simulink model "PURE_PURSUIT"  (R2022b)
settings: Solver=FixedStepAuto  StartTime=0.0  StopTime=400  FixedStep=0.1  RelTol=1e-3
InitFcn:
  | load('pure_pursuit_trajectory.mat');
values from neighbouring files (symbols this model uses):
  trajectory_matrix = trajectory_points    [MAIN_PURE_PURSUIT.m]
undefined symbols (not defined in the file or in its folder): debug_enabled
libraries: robotmobilelib x1
settings Model: Creator=emanuela  LastModifiedBy=emanuela
settings DataIOCC: ReturnWorkspaceOutputs=off

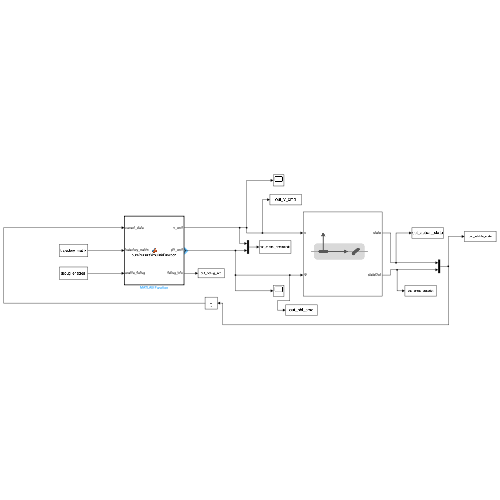
[thumbnail: Simulink's stored preview of the top-level diagram]
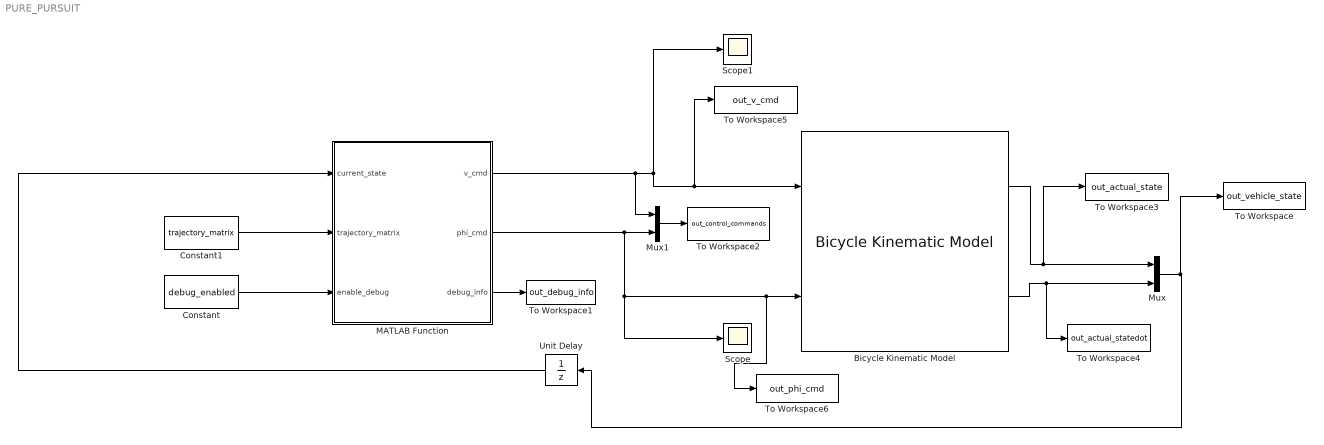
== system PURE_PURSUIT ==
  Bicycle Kinematic Model : robotmobilelib/Bicycle Kinematic Model  VehicleInputs=Vehicle Speed & Steering Angle  WheelBase=2.8  VehicleSpeedRange=[0 3]  MaxSteeringAngle=pi/4  InitialState=initialPose  SimulateUsing=Interpreted execution
  Constant : Constant  Value=debug_enabled
  Constant1 : Constant  Value=trajectory_matrix
  MATLAB Function : MATLAB Function  TreatAsAtomicUnit=on
  Mux : Mux  Inputs=2
  Mux1 : Mux  Inputs=2
  Scope : Scope
  Scope1 : Scope
  To Workspace : ToWorkspace  VariableName=out_vehicle_state  SaveFormat=Timeseries  SampleTime=-1
  To Workspace1 : ToWorkspace  VariableName=out_debug_info  SaveFormat=Timeseries  SampleTime=-1
  To Workspace2 : ToWorkspace  VariableName=out_control_commands  SaveFormat=Timeseries  SampleTime=-1
  To Workspace3 : ToWorkspace  VariableName=out_actual_state  SaveFormat=Timeseries  SampleTime=-1
  To Workspace4 : ToWorkspace  VariableName=out_actual_statedot  SaveFormat=Timeseries  SampleTime=-1
  To Workspace5 : ToWorkspace  VariableName=out_v_cmd  SaveFormat=Timeseries  SampleTime=-1
  To Workspace6 : ToWorkspace  VariableName=out_phi_cmd  SaveFormat=Timeseries  SampleTime=-1
  Unit Delay : UnitDelay  InitialCondition=[36.35,44.05,0,0,0,0]  SampleTime=0.1  HasFrameUpgradeWarning=on
  wires:
  MATLAB Function/2(phi_cmd) -> Mux1/2, Scope/1, To Workspace6/1, Bicycle Kinematic Model/2
  MATLAB Function/1(v_cmd) -> Mux1/1, To Workspace5/1, Bicycle Kinematic Model/1, Scope1/1
  Bicycle Kinematic Model/1 -> To Workspace3/1, Mux/1
  Bicycle Kinematic Model/2 -> To Workspace4/1, Mux/2
  Constant1/1 -> MATLAB Function/2(trajectory_matrix)
  Mux/1 -> To Workspace/1, Unit Delay/1
  Constant/1 -> MATLAB Function/3(enable_debug)
  MATLAB Function/3(debug_info) -> To Workspace1/1
  Mux1/1 -> To Workspace2/1
  Unit Delay/1 -> MATLAB Function/1(current_state)

== matlab function PURE_PURSUIT/MATLAB Function ==
  settings: updateMethod=DISCRETE  sampleTime=0.1
  data: current_state input; v_cmd output; trajectory_matrix input; enable_debug input boolean size=[1 1]; phi_cmd output; debug_info output
function [v_cmd, phi_cmd, debug_info] = purePursuitSimulinkFunction(current_state, trajectory_matrix, enable_debug)
%% ===================================================================
%% OUTPUT INITIALISATION
%% ===================================================================

v_cmd = 0.0;
phi_cmd = 0.0;
debug_info = zeros(1, 8);

%% ===================================================================
%% INPUT VALIDATION
%% ===================================================================

if isempty(current_state) || length(current_state) < 3
    debug_info(1) = -1;
    return;
end

if isempty(trajectory_matrix) || size(trajectory_matrix, 1) < 2 || size(trajectory_matrix, 2) < 3
    debug_info(1) = -2;
    return;
end

persistent parking_complete v_cmd_prev phi_cmd_prev
persistent wheelbase lookahead_distance lookahead_time lookahead_min lookahead_max
persistent v_max v_min phi_max kp_longitudinal
persistent enable_smoothing smoothing_factor
persistent parking_position_threshold parking_angle_threshold parking_velocity_threshold
persistent approach_distance final_approach_v_max alignment_distance alignment_v_max
persistent time_at_goal
persistent startup_counter 
persistent v_des_prev  

if isempty(parking_complete)
    % Stati
    parking_complete = false;
    v_cmd_prev = 0.0;
    phi_cmd_prev = 0.0;
    time_at_goal = 0;
    startup_counter = 0;  
    v_des_prev = 0.0;  
    
    % Parameters
    wheelbase = 2.8;
    lookahead_distance = 4.0;
    lookahead_time = 1.5;
    lookahead_min = 2.0;
    lookahead_max = 15.0;
    
    % Constraints
    v_max = 3.0;
    v_min = 0.0;
    phi_max = pi/4;
    
    % Control
    kp_longitudinal = 0.8;
    enable_smoothing = true;
    smoothing_factor = 0.7;
    
    % Parking 
    parking_position_threshold = 0.08;    
    parking_angle_threshold = 0.02;      
    parking_velocity_threshold = 0.03;    
    approach_distance = 3.0;
    final_approach_v_max = 0.4;
    alignment_distance = 1.0;
    alignment_v_max = 0.2;              
end

startup_counter = startup_counter + 1;

%% ===================================================================
%% CHECK PARKING COMPLETED
%% ===================================================================

if parking_complete
    v_cmd = 0.0;
    phi_cmd = 0.0;
    if enable_debug
        debug_info = [0, 0, 0, 0, 0, 999, 0, 0];
    end
    return;
end

%% ===================================================================
%% STATE 
%% ===================================================================

x_current = current_state(1);
y_current = current_state(2);
theta_current = current_state(3);

if length(current_state) >= 4
    v_current = current_state(4);
else
    v_current = 0.0;  % MODIFICATO: default a 0 invece di 1
end

%% ===================================================================
%% FINAL GOAL 
%% ===================================================================

n_points = size(trajectory_matrix, 1);

% Coordinates final goal
final_x = trajectory_matrix(n_points, 1);
final_y = trajectory_matrix(n_points, 2);
if size(trajectory_matrix, 2) >= 3
    final_theta = trajectory_matrix(n_points, 3);
else
    final_theta = 0.0;
end

% Distance from the goal
dx_goal = final_x - x_current;
dy_goal = final_y - y_current;
dist_to_goal = sqrt(dx_goal*dx_goal + dy_goal*dy_goal);
angle_to_goal = atan2(dy_goal, dx_goal);
angle_error = wrapToPi(final_theta - theta_current);

%% ===================================================================
%% FIND NEAREST POINT
%% ===================================================================

min_distance = inf;
closest_index = 1;
for i = 1:n_points
    dx = trajectory_matrix(i, 1) - x_current;
    dy = trajectory_matrix(i, 2) - y_current;
    dist = sqrt(dx*dx + dy*dy);
    if dist < min_distance
        min_distance = dist;
        closest_index = i;
    end
end

%% ===================================================================
%% COMPLETION CHECK
%% ===================================================================

position_ok = dist_to_goal < parking_position_threshold;
angle_ok = abs(angle_error) < parking_angle_threshold;
velocity_ok = abs(v_current) < parking_velocity_threshold;

if position_ok && angle_ok && velocity_ok
    time_at_goal = time_at_goal + 1;
    if time_at_goal > 10  
        parking_complete = true;
        v_cmd = 0.0;
        phi_cmd = 0.0;
        return;
    end
else
    time_at_goal = 0;
end

remaining = n_points - closest_index;

is_final_phase = dist_to_goal < 0.3;        
is_approach = dist_to_goal < approach_distance && ~is_final_phase;
is_alignment = dist_to_goal < alignment_distance && ~is_final_phase;
is_startup = startup_counter <= 50;  

%% ===================================================================
%% LOOKAHEAD CALCULATION FOR FINAL PHASE
%% ===================================================================

ld = lookahead_distance + abs(v_current) * lookahead_time;

if is_final_phase
    ld = 0.0; 
elseif is_alignment
    ld = max(0.3, min(0.8, dist_to_goal * 0.6));
elseif is_approach
    ld = max(1.0, min(2.0, dist_to_goal * 0.7));
else
    ld = max(lookahead_min, min(lookahead_max, ld));
end

%% ===================================================================
%% TARGET SEARCH 
%% ===================================================================

% If in the final phase OR very close, aim for the correct goal
if is_final_phase || dist_to_goal < 1.0 || closest_index > n_points - 10
    target_index = n_points;
    target_x = final_x;
    target_y = final_y;
else
    
    target_index = closest_index;
    target_x = trajectory_matrix(closest_index, 1);
    target_y = trajectory_matrix(closest_index, 2);
    
    
    for i = closest_index:n_points
        dx = trajectory_matrix(i, 1) - x_current;
        dy = trajectory_matrix(i, 2) - y_current;
        dist = sqrt(dx*dx + dy*dy);
        
        if dist >= ld
            target_index = i;
            target_x = trajectory_matrix(i, 1);
            target_y = trajectory_matrix(i, 2);
            break;
        end
    end
    
   
    if target_index == closest_index && remaining < 20
        target_index = n_points;
        target_x = final_x;
        target_y = final_y;
    end
end

%% ===================================================================
%% STEERING CALCULATION
%% ===================================================================


if is_final_phase
    dx = final_x - x_current;
    dy = final_y - y_current;
    dist_target = dist_to_goal;
else
    dx = target_x - x_current;
    dy = target_y - y_current;
    dist_target = sqrt(dx*dx + dy*dy);
end

alpha = atan2(dy, dx) - theta_current;
alpha = wrapToPi(alpha);


if dist_target > 0.01  
    if is_final_phase
        k = 3.0;  
    elseif is_alignment
        k = 2.0;
    elseif is_approach
        k = 1.5;
    else
        k = 1.0;
    end
    
    phi_cmd = atan(k * 2 * wheelbase * sin(alpha) / dist_target);
else
    phi_cmd = 0.0;
end

phi_cmd = max(-phi_max, min(phi_max, phi_cmd));

if size(trajectory_matrix, 2) >= 4 && target_index <= n_points
    v_des_wp = trajectory_matrix(target_index, 4);
else
    v_des_wp = 0.0;  
end

if is_startup
    
    startup_factor = min(1.0, startup_counter / 50.0);
    
    startup_factor = startup_factor * startup_factor;
    v_des_startup = 0.5 * startup_factor;  
else
    v_des_startup = inf;  
end


if is_final_phase
    
    if dist_to_goal > 0.25
        v_des = 0.15;  
    else
        
        v_des = 0.15 * exp(-10 * (0.25 - dist_to_goal));
        
        if dist_to_goal > parking_position_threshold
            v_des = max(0.02, v_des);
        else
            v_des = 0.0;  
        end
    end
elseif is_alignment
    
    v_des = min(alignment_v_max, 0.05 + 0.15 * sqrt(dist_to_goal));
elseif is_approach
    
    v_des = min(final_approach_v_max, 0.1 + 0.3 * dist_to_goal / approach_distance);
else
    v_des = v_des_wp;
    if abs(phi_cmd) > pi/6
        v_des = v_des * 0.7;
    end
end


v_des = min(v_des, v_des_startup);

if isempty(v_des_prev)
    v_des_prev = 0.0;
end

max_v_change = 0.02;  
if is_final_phase || is_alignment
    max_v_change = 0.01;  
end

v_des_change = v_des - v_des_prev;
if abs(v_des_change) > max_v_change
    v_des = v_des_prev + sign(v_des_change) * max_v_change;
end
v_des_prev = v_des;

% Control with adaptive gain
if is_startup
    kp = kp_longitudinal * 0.3;  
elseif is_final_phase
    
    kp = kp_longitudinal * 0.1 * min(1.0, dist_to_goal / 0.3);
elseif is_alignment
    kp = kp_longitudinal * 0.3;  
elseif is_approach
    kp = kp_longitudinal * 0.5;  
else
    kp = kp_longitudinal;
end

v_err = v_des - v_current;


if is_final_phase || is_alignment
    max_v_err = 0.1;  
    v_err = max(-max_v_err, min(max_v_err, v_err));
end

v_cmd = v_current + kp * v_err;

% VELOCITY LIMITS
v_cmd = max(v_min, min(v_max, v_cmd));


if is_startup
    v_cmd = min(v_cmd, v_des_startup);
end


if ~is_startup && dist_to_goal > parking_position_threshold * 2 && v_cmd < 0.02
    v_cmd = 0.02; 
end


if dist_to_goal < parking_position_threshold * 1.5
    decay_factor = dist_to_goal / (parking_position_threshold * 1.5);
    v_cmd = v_cmd * decay_factor;
end


if enable_smoothing && ~is_final_phase
    if is_startup
        alpha_s = 0.95;  
    elseif is_alignment
        alpha_s = 0.9; 
    elseif is_approach
        alpha_s = 0.85;
    else
        alpha_s = smoothing_factor;
    end
    
    v_cmd = alpha_s * v_cmd + (1 - alpha_s) * v_cmd_prev;
    phi_cmd = alpha_s * phi_cmd + (1 - alpha_s) * phi_cmd_prev;
    
    v_cmd_prev = v_cmd;
    phi_cmd_prev = phi_cmd;
else
    
    if is_final_phase
        alpha_s = 0.92; 
        v_cmd = alpha_s * v_cmd + (1 - alpha_s) * v_cmd_prev;
        phi_cmd = alpha_s * phi_cmd + (1 - alpha_s) * phi_cmd_prev;
    end
    
   
    v_cmd_prev = v_cmd;
    phi_cmd_prev = phi_cmd;
end

if enable_debug
    debug_info(1) = dist_to_goal;
    debug_info(2) = dist_target;
    debug_info(3) = ld;
    debug_info(4) = phi_cmd;
    debug_info(5) = v_err;
    debug_info(6) = target_index;
    debug_info(7) = alpha;
    debug_info(8) = v_des;
end

end

function angle = wrapToPi(angle)
    while angle > pi
        angle = angle - 2*pi;
    end
    while angle < -pi
        angle = angle + 2*pi;
    end
end
